simulink model "frenagem_real"  (R2016a)
settings: Solver=ode45  StartTime=0.0  StopTime=50  FixedStep=.03  MinStep=.04  RelTol=1
libraries: dspvision x2
settings Model: Creator=vmaraccini  LastModifiedBy=vmaraccini-personal
settings DataIOCC: LimitDataPoints=on  SaveFormat=Array
settings HardwareCC: ProdBitPerPointer=32  ProdLargestAtomicFloat=None  ProdIntDivRoundTo=Undefined  ProdEndianess=Unspecified  ProdWordSize=32  ProdHWDeviceType=32-bit Generic
settings ModelReferenceCC: PropagateSignalLabelsOutOfModel=off
settings ConfigComp: CovModelRefEnable=Off

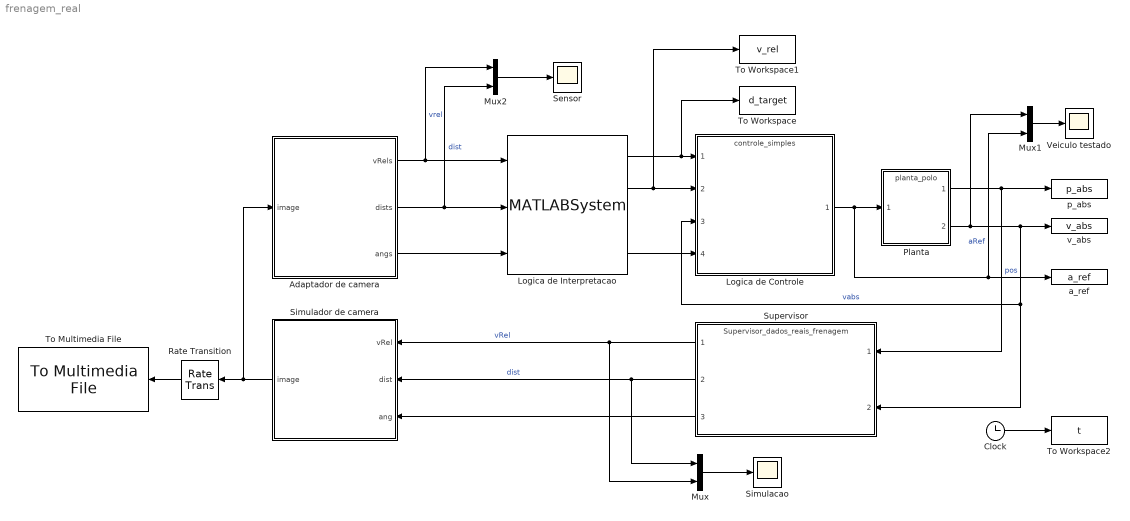
== system frenagem_real ==
  Adaptador de camera : Subsystem
  Clock : Clock
  Logica de Controle : ModelReference  ModelNameDialog=controle_simples.slx  SimulationMode=Normal  ModelReferenceVersion=1.108
  Logica de Interpretacao : MATLABSystem  System=Interpretacao  SimulateUsing=Interpreted execution
      mask Type: Interpretacao
      mask Display:
      | disp('Interpretacao');
      | port_label('input',1,'vrels');
      | port_label('input',2,'dists');
      | port_label('input',3,'angs');
      | port_label('output',1,'dist');
      | port_label('output',2,'vrel');
      | port_label('output',3,'ang');
      | port_label('output',4,'vmax');
  Mux : Mux  Inputs=2
  Mux1 : Mux  Inputs=2
  Mux2 : Mux  Inputs=2
  Planta : ModelReference  ModelNameDialog=planta_polo.slx  SimulationMode=Normal  ModelReferenceVersion=1.1
  Rate Transition : RateTransition  OutPortSampleTime=.0416
  Sensor : Scope
  Simulacao : Scope
  Simulador de camera : Subsystem
  Supervisor : ModelReference  ModelNameDialog=Supervisor_dados_reais_frenagem.slx  SimulationMode=Normal  ModelReferenceVersion=1.3
  To Multimedia File : dspvision/To Multimedia File  outputFilename=camera_sim.avi  streamSelection=Video only  videoCompressor=MJPEG Compressor  audioCompressor=None (uncompressed)  imagePorts=One multidimensional signal  fileType=AVI  audioDatatype=Determine from input data type  fourcc=RGB  videoQuality=75  mj2000CompFactor=10
  To Workspace : ToWorkspace  VariableName=d_target  SampleTime=-1
      settings: Save2DSignal=2-D array (concatenate along first dimension)
  To Workspace1 : ToWorkspace  VariableName=v_rel  SampleTime=-1
      settings: Save2DSignal=2-D array (concatenate along first dimension)
  To Workspace2 : ToWorkspace  VariableName=t  SampleTime=-1
      settings: Save2DSignal=2-D array (concatenate along first dimension)
  Veiculo testado : Scope
  a_ref : ToWorkspace  VariableName=a_ref  SampleTime=-1
      settings: Save2DSignal=2-D array (concatenate along first dimension)
  p_abs : ToWorkspace  VariableName=p_abs  SampleTime=-1
      settings: Save2DSignal=2-D array (concatenate along first dimension)
  v_abs : ToWorkspace  VariableName=v_abs  SampleTime=-1
      settings: Save2DSignal=2-D array (concatenate along first dimension)
  wires:
  Planta/2 -> Supervisor/2, Logica de Controle/3, v_abs/1, Mux1/1  "vabs"
  Logica de Controle/1 -> Planta/1, Mux1/2, a_ref/1  "aRef"
  Planta/1 -> Supervisor/1, p_abs/1  "pos"
  Logica de Interpretacao/1 -> To Workspace/1, Logica de Controle/1
  Supervisor/1 -> Mux/2, Simulador de camera/1(vRel)  "vRel"
  Supervisor/2 -> Mux/1, Simulador de camera/2(dist)  "dist"
  Mux/1 -> Simulacao/1
  Mux1/1 -> Veiculo testado/1
  Logica de Interpretacao/4 -> Logica de Controle/4
  Logica de Interpretacao/2 -> Logica de Controle/2, To Workspace1/1
  Adaptador de camera/3(angs) -> Logica de Interpretacao/3
  Adaptador de camera/1(vRels) -> Mux2/1, Logica de Interpretacao/1  "vrel"
  Adaptador de camera/2(dists) -> Mux2/2, Logica de Interpretacao/2  "dist"
  Mux2/1 -> Sensor/1
  Clock/1 -> To Workspace2/1
  Rate Transition/1 -> To Multimedia File/1
  Simulador de camera/1(image) -> Adaptador de camera/1(image), Rate Transition/1
  Supervisor/3 -> Simulador de camera/3(ang)

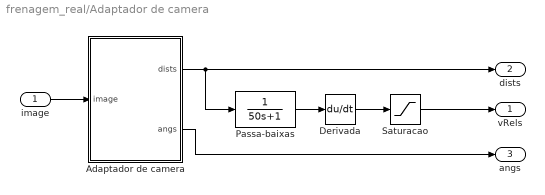
== system frenagem_real/Adaptador de camera ==
  image : Inport
  Adaptador de camera : MATLAB Function  TreatAsAtomicUnit=on
  Derivada : Derivative
  Passa-baixas : TransferFcn  Numerator=1  Denominator=[50 1]
  Saturacao : Saturate  UpperLimit=100  LowerLimit=-10
  vRels : Outport
  dists : Outport  Port=2
  angs : Outport  Port=3
  wires:
  image/1 -> Adaptador de camera/1(image)
  Adaptador de camera/1(dists) -> Passa-baixas/1, dists/1
  Adaptador de camera/2(angs) -> angs/1
  Derivada/1 -> Saturacao/1
  Saturacao/1 -> vRels/1
  Passa-baixas/1 -> Derivada/1

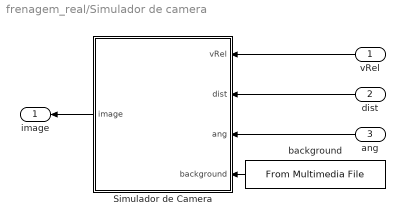
== system frenagem_real/Simulador de camera ==
  vRel : Inport
  dist : Inport  Port=2
  ang : Inport  Port=3
  Simulador de Camera : MATLAB Function  TreatAsAtomicUnit=on
  background : dspvision/From Multimedia File  inputFilename=/Users/vmaraccini-personal/Documents/MATLAB/TCC/camera/camera_template.avi  loop=on  numPlays=inf  outputStreams=Video only  videoDataType=uint8  audioDataType=int16  inheritSampleTime=on  userDefinedSampleTime=1/30  noAudioOutput=off  isIntensityVideo=off  fourcc=Intensity  colorVideoFormat=One multidimensional signal  outputEOF=off  dataOrg=Column-major  audioFrameSize=1024  computeAudioFrameSize=off  outSamplingMode=Sample based
  image : Outport
  wires:
  ang/1 -> Simulador de Camera/3(ang)
  Simulador de Camera/1(image) -> image/1
  dist/1 -> Simulador de Camera/2(dist)
  vRel/1 -> Simulador de Camera/1(vRel)
  background/1 -> Simulador de Camera/4(background)

== matlab function frenagem_real/Simulador de camera/Simulador de Camera ==
  data: vRel input; image output; dist input; ang input; background input
function image = simula_camera(vRel, dist, ang, background)
imgSize = 200;
dMax = 50;

image = uint8(zeros(imgSize, imgSize));

image = background;
% image = imresize(road_template, [imgSize, imgSize]);

% Adicionar ruido simulando fundo
image = image + uint8(255*rand(imgSize)/10); %10% de dMax

% Adicionar carro
if dist < 1
    dist = 1;
end
if dist > dMax
    dist = dMax;
end

% Adicionar ruido branco sobre o carro
tamanho = ceil(imgSize*.5*(1-dist/dMax));
tamanhoW = round(tamanho);
tamanhoH = round(0.7*tamanho);
displace = 15;

carro = rand(tamanhoH, tamanhoW)*0.1*(dist/dMax);
carro = carro + dist/dMax * ones(tamanhoH, tamanhoW);

image((end/2 - ceil(tamanhoH/2) + displace + 1) : (end/2 + floor(tamanhoH/2) + displace), ...
    (end/2 - ceil(tamanhoW/2) + 1) : end/2 + floor(tamanhoW/2)) = ...
    uint8(255*(1-carro));

end

== matlab function frenagem_real/Adaptador de camera/Adaptador de camera ==
  data: image input; dists output; angs output
function [dists, angs] = fcn(image)
numVehicles = 1;
dMax = 50;

dists = zeros(1,numVehicles);
angs = zeros(1,numVehicles);

dists = ones(1, numVehicles) * (1 - double(image(end/2,end/2))/255) * dMax;
angs = zeros(1, numVehicles);

end
